simulink model "hw3_problem4"  (R2016a)
settings: Solver=VariableStepAuto  StartTime=0  StopTime=5  RelTol=1e-3
values from neighbouring files (symbols this model uses):
  bu_tot = 1    [hw3.m]
  f_d = 0    [hw3.m]
  kx_l = 0    [hw3.m]
  L = 1e-3    (= 0.001)    [hw3.m]
  Lambda_pm0oell = 1    [hw3.m]
  m_tot = 10e3    (= 10000)    [hw3.m]
  R = 100e-3    (= 0.1)    [hw3.m]
  V_bus = 5    [hw3.m]
libraries: cstblocks x1
settings Model: Creator=Seth Barger  LastModifiedBy=Seth Barger

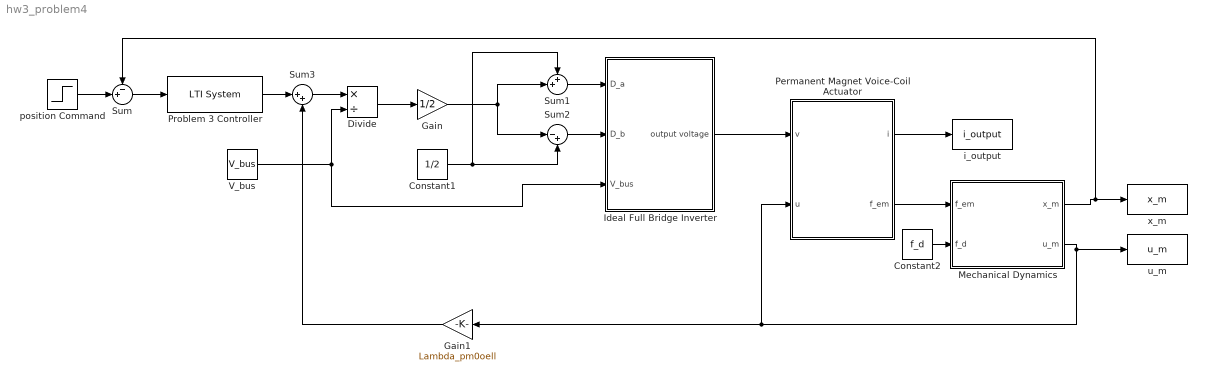
== system hw3_problem4 ==
  Constant1 : Constant  Value=1/2
  Constant2 : Constant  Value=f_d
  Divide : Product  Inputs=*/
  Gain : Gain  Gain=1/2
  Gain1 : Gain  Gain=Lambda_pm0oell
  "Ideal Full Bridge Inverter " : Subsystem
  Mechanical Dynamics : Subsystem
  Permanent Magnet Voice-Coil Actuator : Subsystem
  Problem 3 Controller : cstblocks/LTI System  sys=Gtot  IC=[]
  Sum : Sum  Inputs=-+|
  Sum1 : Sum  Inputs=++|
  Sum2 : Sum  Inputs=|-+
  Sum3 : Sum  Inputs=|++
  V_bus : Constant  Value=V_bus
  i_output : ToWorkspace  VariableName=i_output  SampleTime=-1
  "position Command " : Step  Time=0  After=.01  SampleTime=0
  u_m : ToWorkspace  VariableName=u_m  SampleTime=-1
  x_m : ToWorkspace  VariableName=x_m  SampleTime=-1
  wires:
  "Ideal Full Bridge Inverter "/1(output voltage) -> Permanent Magnet Voice-Coil Actuator/1(v)
  Sum/1 -> Problem 3 Controller/1
  "position Command "/1 -> Sum/2
  Permanent Magnet Voice-Coil Actuator/1(i) -> i_output/1
  Divide/1 -> Gain/1
  Gain/1 -> Sum2/1, Sum1/2
  Constant1/1 -> Sum1/1, Sum2/2
  V_bus/1 -> "Ideal Full Bridge Inverter "/3(V_bus), Divide/2
  Sum1/1 -> "Ideal Full Bridge Inverter "/1(D_a)
  Sum2/1 -> "Ideal Full Bridge Inverter "/2(D_b)
  Permanent Magnet Voice-Coil Actuator/2(f_em) -> Mechanical Dynamics/1(f_em)
  Mechanical Dynamics/2(u_m) -> u_m/1, Permanent Magnet Voice-Coil Actuator/2(u), Gain1/1
  Constant2/1 -> Mechanical Dynamics/2(f_d)
  Mechanical Dynamics/1(x_m) -> x_m/1, Sum/1
  Sum3/1 -> Divide/1
  Problem 3 Controller/1 -> Sum3/1
  Gain1/1 -> Sum3/2

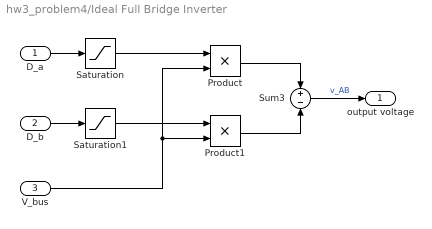
== system hw3_problem4/Ideal Full Bridge Inverter  ==
  D_a : Inport
  D_b : Inport  Port=2
  V_bus : Inport  Port=3
  Product : Product
  Product1 : Product
  Saturation : Saturate  UpperLimit=1  LowerLimit=0
  Saturation1 : Saturate  UpperLimit=1  LowerLimit=0
  Sum3 : Sum  Inputs=+-  SaturateOnIntegerOverflow=on
  output voltage : Outport
  wires:
  Sum3/1 -> output voltage/1  "v_AB"
  D_a/1 -> Saturation/1
  D_b/1 -> Saturation1/1
  V_bus/1 -> Product1/2, Product/2
  Product/1 -> Sum3/1
  Product1/1 -> Sum3/2
  Saturation/1 -> Product/1
  Saturation1/1 -> Product1/1

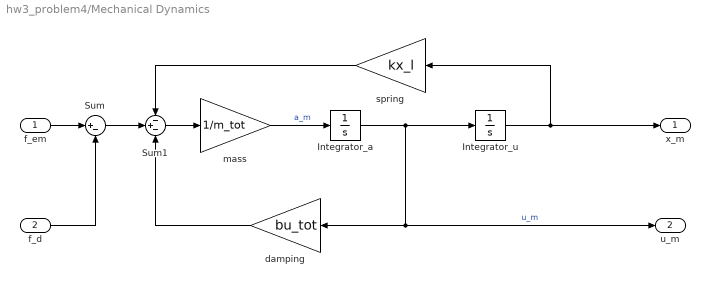
== system hw3_problem4/Mechanical Dynamics ==
  f_em : Inport
  f_d : Inport  Port=2
  Integrator_a : Integrator
  Integrator_u : Integrator
  Sum : Sum  Inputs=|+-
  Sum1 : Sum  Inputs=-+-
  damping : Gain  Gain=bu_tot
  mass : Gain  Gain=1/m_tot
  spring : Gain  Gain=kx_l
  x_m : Outport
  u_m : Outport  Port=2
  wires:
  f_em/1 -> Sum/1
  f_d/1 -> Sum/2
  mass/1 -> Integrator_a/1  "a_m"
  Integrator_a/1 -> Integrator_u/1, u_m/1, damping/1  "u_m"
  Integrator_u/1 -> x_m/1, spring/1
  Sum/1 -> Sum1/2
  Sum1/1 -> mass/1
  damping/1 -> Sum1/3
  spring/1 -> Sum1/1

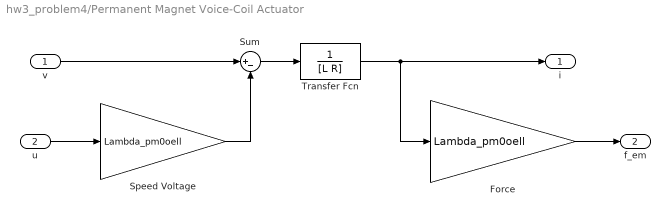
== system hw3_problem4/Permanent Magnet Voice-Coil Actuator ==
  v : Inport
  u : Inport  Port=2
  Force : Gain  Gain=Lambda_pm0oell
  Speed Voltage : Gain  Gain=Lambda_pm0oell
  Sum : Sum  Inputs=|+-
  Transfer Fcn : TransferFcn  Denominator=[L R]
  i : Outport
  f_em : Outport  Port=2
  wires:
  Transfer Fcn/1 -> i/1, Force/1
  Force/1 -> f_em/1
  v/1 -> Sum/1
  u/1 -> Speed Voltage/1
  Speed Voltage/1 -> Sum/2
  Sum/1 -> Transfer Fcn/1
